simulink model "Ld_Lq_realised_inverter"  (R2024a)
settings: Solver=ode23tb  StartTime=0.0  StopTime=0.25  MaxStep=1e-7  RelTol=1e-3  EnableMultiTasking=on
undefined symbols (not defined in the file): sigbuilder_block
libraries: spsSeriesRLCBranchLib x8, spsVoltageMeasurementLib x8, spsIGBTDiodeLib x6, spsRMSLib x4, spsCurrentMeasurementLib x3, spsMeanLib x3, simulink x3, spsPermanentMagnetSynchronousMachineLib x1, spsThreePhaseSourceLib x1, spsUniversalBridgeLib x1, spspowerguiLib x1
settings Model: Creator=Алексей  LastModifiedBy=alexey
settings SolverCC: ZeroCrossControl=DisableAll  ZeroCrossAlgorithm=Adaptive  AlgebraicLoopSolver=TrustRegion
settings DataIOCC: SaveFormat=Array  SaveOutput=off  SignalLogging=off  DSMLogging=off  SaveTime=off  ReturnWorkspaceOutputs=off
settings OptimizationCC: LifeSpan=inf
settings DebuggingCC: UnderspecifiedInitializationDetection=Classic  MergeDetectMultiDrivingBlocksExec=none  SolverPrmCheckMsg=warning  UnconnectedInputMsg=warning  UnconnectedOutputMsg=warning  UnconnectedLineMsg=warning  AllowSymbolicDim=off  SFUnexpectedBacktrackingDiag=warning  SFNoUnconditionalDefaultTransitionDiag=warning  SFExecutionAtInitializationDiag=none  ArithmeticOperatorsInVariantConditions=warning
settings HardwareCC: ProdBitPerPointer=32  ProdBitPerSizeT=32  ProdBitPerPtrDiffT=32  ProdLargestAtomicFloat=None  ProdIntDivRoundTo=Undefined  ProdEndianess=Unspecified  ProdWordSize=32  ProdHWDeviceType=32-bit Generic
settings ModelReferenceCC: EnableRefExpFcnMdlSchedulingChecks=on  PropagateSignalLabelsOutOfModel=off
settings SFSimCC: SimUseLocalCustomCode=off  CustomCodeUndefinedFunction=UseInterfaceOnly
settings RTWCC: RTWUseLocalCustomCode=off  GPUComputeCapability=3.5  DLArmComputeVersion=19.05
settings CodeAppCC: StateflowObjectComments=on
settings GRTTargetCC: TargetLangStandard=C89/C90 (ANSI)  RTWCAPISignals=on  RTWCAPIParams=on
settings ConfigComp: CovMetricSettings=dw  CovSaveCumulativeToWorkspaceVar=on  CovSaveSingleToWorkspaceVar=on  CovExternalEMLEnable=off  CovSFcnEnable=off
settings SimscapeCC: SimscapeNormalizeSystem=off

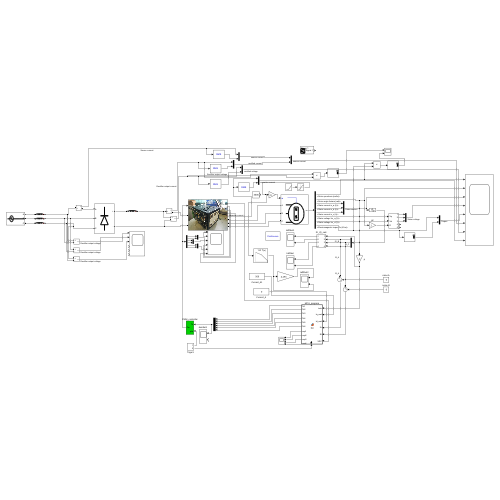
[thumbnail: Simulink's stored preview of the top-level diagram]
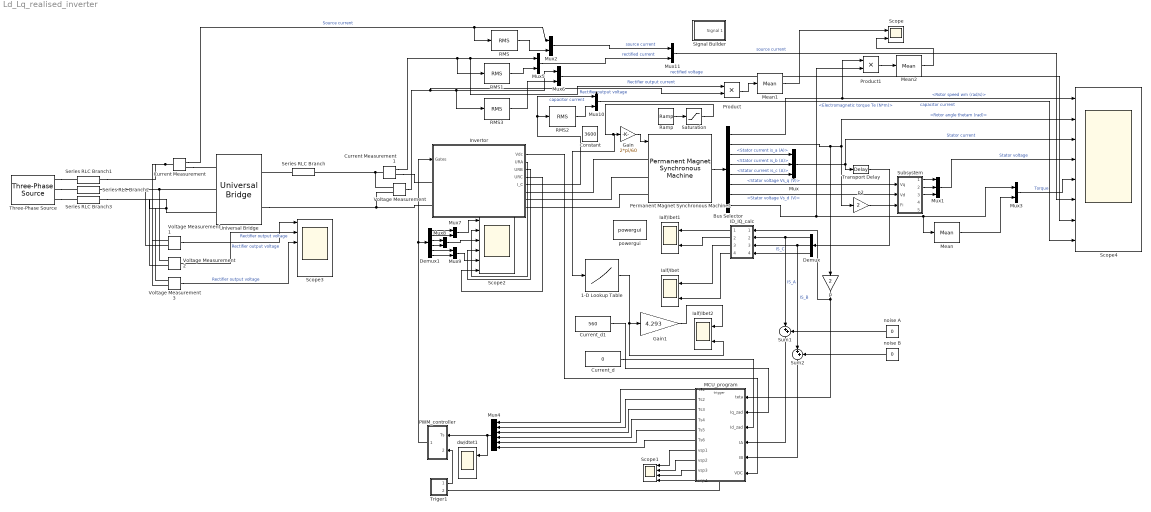
== system Ld_Lq_realised_inverter ==
  1-D Lookup Table : Lookup_n-D  NumberOfTableDimensions=1  BreakpointsForDimension1=[0 2834 5667 5668 5669]  Table=[140 105 25 0 0]  InternalRulePriority=Speed  RndMeth=Simplest
  Bus Selector : BusSelector  OutputSignals=Rotor speed wm (rad/s),Rotor angle thetam (rad),Stator current is_a (A),Stator current is_b (A),Stator current is_c (A),Stator voltage Vs_q (V),Stator voltage Vs_d (V),Electromagnetic torque Te (N*m)
  Constant : Constant  Value=3600
  Current Measurement : spsCurrentMeasurementLib/Current Measurement  PhasorSimulation=off  OutputType=Complex  PSBequivalent=0
  Current Measurement1 : spsCurrentMeasurementLib/Current Measurement  PhasorSimulation=off  OutputType=Complex  PSBequivalent=0
  Current_d : Constant  Value=0
  Current_d1 : Constant  Value=560
  Demux : Demux  Outputs=3
  Demux1 : Demux  Outputs=6
  Gain : Gain  Gain=2*pi/60
  Gain1 : Gain  Gain=4.293
  ID_IQ_calc : Subsystem
  Ialf/Ibet : Scope  NumInputPorts=2
  Ialf/Ibet1 : Scope  NumInputPorts=2
  Ialf/Ibet2 : Scope  NumInputPorts=2
  Invertor : Subsystem
      mask Display: image('$imagefile'); % Use "Edit Image" on toolstrip to change.
  MCU_program : MATLAB Function  TreatAsAtomicUnit=on
  Mean : spsMeanLib/Mean  Freq=1000  Vinit=0  Ts=0
  Mean1 : spsMeanLib/Mean  Freq=400  Vinit=0  Ts=0
  Mean2 : spsMeanLib/Mean  Freq=400  Vinit=0  Ts=0
  Mux : Mux  Inputs=3
  Mux1 : Mux  Inputs=3
  Mux{2..3,5..11} (9 alike) : Mux  Inputs=2
  Mux4 : Mux  Inputs=6
  PWM_controller : Subsystem
  Permanent Magnet Synchronous Machine1 : spsPermanentMagnetSynchronousMachineLib/Permanent Magnet Synchronous Machine  NbPhases=3  FluxDistribution=Sinusoidal  RotorType=Round  MechanicalLoad=Speed w  PresetModel=No  ShowDetailedParameters=on  MeasurementBus=off  Resistance=0.00285  Inductance=8.5e-3  dqInductances=[0.37e-3, 1.075e-3]  La=68.03e-6  MachineConstant=Flux linkage established by magnets (V.s)  Flux=0.07763  VoltageCst=28.161  TorqueCst=0.23289  Flat=120  Mechanical=[2e104 3e-03 2 0]  PolePairs=2  InitialConditions=[0,0, 0,0]  InitialConditions5ph=[0 0 0 0 0 0]  RefAngle=Aligned with phase A axis (original Park)  IterativeDiscreteModel=Trapezoidal non iterative  TsBlock=-1  TsPowergui=0
  Product : Product
  Product1 : Product
  RMS : spsRMSLib/RMS  TrueRMS=on  Freq=400  RMSInit=120  Ts=0
  RMS1 : spsRMSLib/RMS  TrueRMS=on  Freq=400  RMSInit=120  Ts=0
  RMS2 : spsRMSLib/RMS  TrueRMS=on  Freq=400  RMSInit=120  Ts=0
  RMS3 : spsRMSLib/RMS  TrueRMS=on  Freq=400  RMSInit=280  Ts=0
  Ramp : simulink/Sources/Ramp  slope=36000  start=0.01  InitialOutput=0
  Saturation : Saturate  UpperLimit=5600
  Scope : Scope  NumInputPorts=2
  Scope1 : Scope  NumInputPorts=4
  Scope2 : Scope  NumInputPorts=6
  Scope3 : Scope  NumInputPorts=6
  Scope4 : Scope  NumInputPorts=8
  Series RLC Branch : spsSeriesRLCBranchLib/Series RLC Branch  LConnTagsString=__new0  RConnTagsString=__new0  BranchType=L  Resistance=1  Inductance=15e-6  SetiL0=off  InitialCurrent=0  Capacitance=1000e-6  Setx0=on  InitialVoltage=282  Measurements=None
  Series RLC Branch1 : spsSeriesRLCBranchLib/Series RLC Branch  LConnTagsString=__new0  RConnTagsString=__new0  BranchType=L  Resistance=1  Inductance=50e-9  SetiL0=off  InitialCurrent=0  Capacitance=1000e-6  Setx0=on  InitialVoltage=282  Measurements=None
  Series RLC Branch2 : spsSeriesRLCBranchLib/Series RLC Branch  LConnTagsString=__new0  RConnTagsString=__new0  BranchType=L  Resistance=1  Inductance=50e-9  SetiL0=off  InitialCurrent=0  Capacitance=1000e-6  Setx0=on  InitialVoltage=282  Measurements=None
  Series RLC Branch3 : spsSeriesRLCBranchLib/Series RLC Branch  LConnTagsString=__new0  RConnTagsString=__new0  BranchType=L  Resistance=1  Inductance=50e-9  SetiL0=off  InitialCurrent=0  Capacitance=1000e-6  Setx0=on  InitialVoltage=282  Measurements=None
  Signal Builder : Subsystem  Tag=STV Subsys  LoadFcn=sigbuilder_block('load');  StartFcn=sigbuilder_block('start');  StopFcn=sigbuilder_block('stop');  ClipboardFcn=sigbuilder_block('clipboard');  mask(Sigbuilder block){tuvar=[0:10]}
      mask help: Simulink:masks:SigbuilderBlock_MD
      mask init:
      | if ~strcmp(get_param(bdroot(gcbh),'SimulationStatus'),'stopped') tuvar = sigbuilder_block('maskInit'); end
      settings: CopyFcn=sigbuilder_block('copy');  DeleteFcn=sigbuilder_block('delete');  ModelCloseFcn=sigbuilder_block('modelClose');  PreSaveFcn=sigbuilder_block('preSave');  PauseFcn=sigbuilder_block('pause');  ContinueFcn=sigbuilder_block('continue');  NameChangeFcn=sigbuilder_block('namechange');  OpenFcn=sigbuilder_block('open',[60 199.2 1136.8 400 ]);  CloseFcn=sigbuilder_block('close');
      mask Display: plot(0, 0, 100, 100,[2, 2, 32, 32, 2], [68, 8, 8, 68, 68],[32, 2], [38, 38], [32, 19, 2],[53, 60, 44], [32, 17, 17, 2],[16, 16, 31, 31]);txt = getActiveGroup(gcbh);text(2, 100, txt,'verticalAlignment', 'top');
  Subsystem : Subsystem
  Sum1 : Sum  Inputs=|++
  Sum2 : Sum  Inputs=|++
  Three-Phase Source : spsThreePhaseSourceLib/Three-Phase Source  InternalConnection=Y  VoltagePhases=off  Voltage=200  PhaseAngle=0  Voltage_phases=[25e3 25e3 25e3]/sqrt(3)  PhaseAngles_phases=[0 -120 +120]  Frequency=400  NonIdealSource=off  SpecifyImpedance=off  Resistance=0.02e-3  Inductance=30e-9  ShortCircuitLevel=100e6  BaseVoltage=200  XRratio=7  BusType=swing  Pref=10e3  Qref=0  Prefabc=[10e3, 10e3, 10e3]  Qrefabc=[0, 0, 0]  Qmin=-inf  Qmax=inf
  Transport Delay : TransportDelay  DelayTime=5e-6
  Triger1 : Subsystem
  Universal Bridge : spsUniversalBridgeLib/Universal Bridge  Arms=3  SnubberResistance=1e5  SnubberCapacitance=inf  Device=Diodes  Ron=1e-3  Lon=0  ForwardVoltages="[  0  0  ]"  ForwardVoltage=0  GTOparameters=[ 10e-6 , 20e-6 ]  IGBTparameters=[ 1e-6 , 2e-6 ]  Measurements=None  Measurements_2=None  converterType=Rectifier
  Voltage Measurement{,1..3} (4 alike) : spsVoltageMeasurementLib/Voltage Measurement  PhasorSimulation=off  OutputType=Complex  PSBequivalent=0
  dw/dtet1 : Scope  NumInputPorts=2
  noise A : Constant  Value=0
  noise B : Constant  Value=0
  p : Gain  Gain=2
  p2 : Gain  Gain=2
  powergui : spspowerguiLib/powergui  Priority=1  SimulationMode=Continuous  SampleTime=50e-6  frequency=60  Iterations=50  frequencyindice=0  Pbase=100e6  ErrMax=1e-4  UnitsV=kV  UnitsW=MW  buscounter=0  FunctionMessages=off  echomessages=off  EnableUseOfTLC=off  CurrentSourceSwitches=on  DisableSnubberDevices=off  DisableRonSwitches=off  DisableVfSwitches=off  DisplayEquations=off  AutomaticDiscreteSolvers=off  SolverType=Tustin  Interpol=off  ExternalGateDelay=off  methode=off  Ts=0  x0status=blocks  SPID=off  SwTol=0  HookPort=off  NonlinearTolerance=1e-4  nMaxIteration=100  ContinueOnMaxIteration=off  RestoreLinks=warning  ResistiveCurrentMeasurement=off  Frange=[0:2:500]  Ylog=off  Xlog=on  ShowGrid=off  save=off  variable=ZData  structure=SD2  ZoomFFT=on  StartTime=0.7  cycles=10  DisplayStyle=4  fundamental=382  FreqAxis=off  MaxFrequency=50000  frequencyindicesteady=1  RmsSteady=1  display=off
  wires:
  Demux/1 -> ID_IQ_calc/2(In2), Sum1/1  "IS_A"
  Demux/2 -> ID_IQ_calc/3(In3), Sum2/1  "IS_B"
  Permanent Magnet Synchronous Machine1/1 -> Bus Selector/1
  Bus Selector/3 -> Mux/1  "<Stator current is_a (A)>"
  Bus Selector/4 -> Mux/2  "<Stator current is_b (A)>"
  Bus Selector/5 -> Mux/3  "<Stator current is_c (A)>"
  Bus Selector/6 -> Subsystem/1(Vq)  "<Stator voltage Vs_q (V)>"
  Bus Selector/7 -> Subsystem/2(Vd)  "<Stator voltage Vs_d (V)>"
  Subsystem/2(Out2) -> Mux1/2
  Subsystem/3(Out3) -> Mux1/3
  Subsystem/1(Out1) -> Mux1/1
  Mux/1 -> Scope4/3, Transport Delay/1  "Stator current"
  Mux1/1 -> Scope4/4  "Stator voltage"
  Bus Selector/8 -> Product1/2, Mean/1, Mux3/1  "<Electromagnetic torque Te (N*m)>"
  Demux/3 -> ID_IQ_calc/4(In4)  "IS_C"
  Gain/1 -> Permanent Magnet Synchronous Machine1/1
  MCU_program/8(vsp2) -> Scope1/2
  MCU_program/9(vsp3) -> Scope1/3
  MCU_program/7(vsp1) -> Scope1/1
  Sum1/1 -> MCU_program/4(IA)
  Sum2/1 -> MCU_program/5(IB)
  Bus Selector/1 -> Product1/1, Scope4/1  "<Rotor speed wm (rad/s)>"
  Bus Selector/2 -> p2/1, Scope4/2, p/1  "<Rotor angle thetam (rad)>"
  Transport Delay/1 -> Demux/1
  noise A/1 -> Sum1/2
  noise B/1 -> Sum2/2
  MCU_program/10(vsp4) -> Scope1/4
  ID_IQ_calc/3(Out3) -> Ialf/Ibet/1
  ID_IQ_calc/4(Out4) -> Ialf/Ibet/2
  p/1 -> MCU_program/1(teta), ID_IQ_calc/1(In1)
  p2/1 -> Subsystem/3(Fi)
  Gain1/1 -> Ialf/Ibet2/1
  Current_d/1 -> MCU_program/3(Id_zad)
  ID_IQ_calc/1(Out1) -> Ialf/Ibet1/1
  ID_IQ_calc/2(Out2) -> Ialf/Ibet1/2
  Mux3/1 -> Scope4/5  "Torque"
  Mean/1 -> Mux3/2
  Demux1/6 -> Mux9/2
  MCU_program/6(Ts6) -> Mux4/6
  MCU_program/5(Ts5) -> Mux4/5
  Demux1/1 -> Mux7/1
  MCU_program/4(Ts4) -> Mux4/4
  Invertor/3(URB) -> Scope2/4
  Demux1/5 -> Mux9/1
  Demux1/4 -> Mux8/2
  MCU_program/3(Ts3) -> Mux4/3
  Triger1/1(1) -> PWM_controller/2(pila)
  Mux9/1 -> Scope2/5
  PWM_controller/1(Tss) -> Invertor/1(Gates), Demux1/1
  Mux7/1 -> Scope2/1
  Demux1/2 -> Mux7/2
  MCU_program/1(Ts1) -> Mux4/1
  Mux4/1 -> dw/dtet1/1, PWM_controller/1(Ts)
  Triger1/2(2) -> MCU_program/Trigger
  MCU_program/2(Ts2) -> Mux4/2
  Invertor/2(URA) -> Scope2/2
  Demux1/3 -> Mux8/1
  Mux8/1 -> Scope2/3
  Invertor/4(URC) -> Scope2/6
  Invertor/1(Vdc) -> MCU_program/6(VDC)
  Invertor/5(I_C) -> RMS2/1, Mux10/1  "capacitor current"
  Current Measurement/1 -> RMS/1, Mux2/1  "Source current"
  Current Measurement1/1 -> RMS1/1, Product/1, Mux5/1  "Rectifier output current"
  Voltage Measurement/1 -> Product/2, RMS3/1, Mux6/1  "Rectifier output voltage"
  Mux2/1 -> Mux11/1  "source current"
  RMS/1 -> Mux2/2
  Mux5/1 -> Mux11/2  "rectified current"
  Mux6/1 -> Scope4/7  "rectified voltage"
  RMS1/1 -> Mux5/2
  RMS2/1 -> Mux10/2
  Mux10/1 -> Scope4/8  "capacitor current"
  RMS3/1 -> Mux6/2
  Saturation/1 -> 1-D Lookup Table/1, Gain/1
  1-D Lookup Table/1 -> Ialf/Ibet2/2, Gain1/1
  Mux11/1 -> Scope4/6  "source current"
  Current_d1/1 -> MCU_program/2(Iq_zad)
  Ramp/1 -> Saturation/1
  Voltage Measurement1/1 -> Scope3/1  "Rectifier output voltage"
  Voltage Measurement2/1 -> Scope3/2  "Rectifier output voltage"
  Voltage Measurement3/1 -> Scope3/3  "Rectifier output voltage"
  Product/1 -> Mean1/1
  Mean1/1 -> Scope/1
  Product1/1 -> Mean2/1
  Mean2/1 -> Scope/2
  connections:
  Permanent Magnet Synchronous Machine1/LConn1 -- Invertor/RConn1
  Permanent Magnet Synchronous Machine1/LConn3 -- Invertor/RConn3
  Permanent Magnet Synchronous Machine1/LConn2 -- Invertor/RConn2
  Current Measurement/LConn1 -- Series RLC Branch1/LConn1 -- Voltage Measurement1/LConn1 -- Voltage Measurement3/LConn2
  Series RLC Branch2/LConn1 -- Voltage Measurement1/LConn2 -- Voltage Measurement2/LConn1 -- Universal Bridge/LConn2
  Series RLC Branch3/LConn1 -- Voltage Measurement2/LConn2 -- Voltage Measurement3/LConn1 -- Universal Bridge/LConn3
  Current Measurement1/RConn1 -- Invertor/LConn1
  Universal Bridge/RConn2 -- Voltage Measurement/LConn2 -- Invertor/LConn2
  Current Measurement/RConn1 -- Universal Bridge/LConn1
  Series RLC Branch/RConn1 -- Universal Bridge/RConn1
  Current Measurement1/LConn1 -- Voltage Measurement/LConn1 -- Series RLC Branch/LConn1
  Three-Phase Source/RConn1 -- Series RLC Branch1/RConn1
  Three-Phase Source/RConn2 -- Series RLC Branch2/RConn1
  Three-Phase Source/RConn3 -- Series RLC Branch3/RConn1

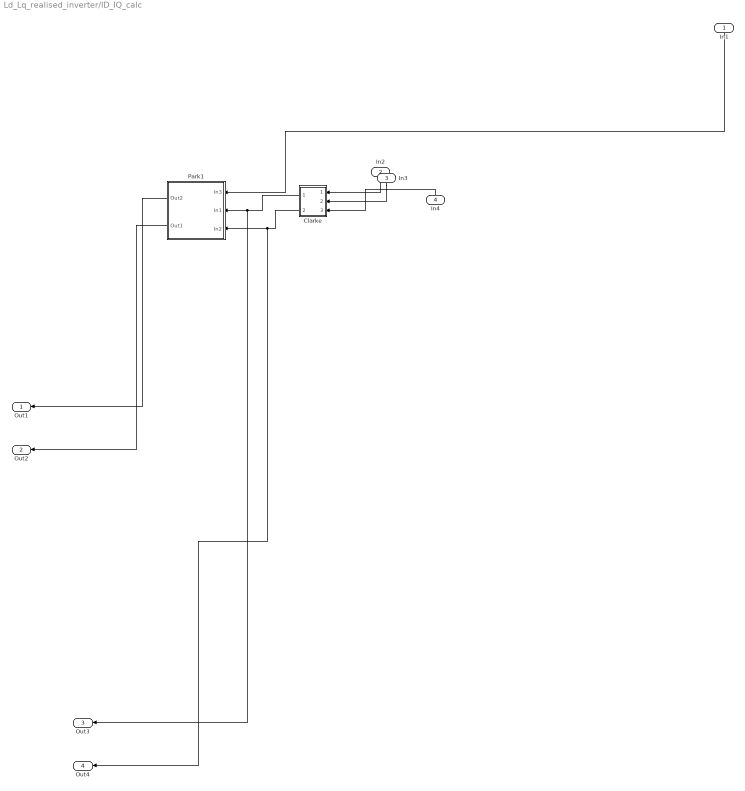
== system Ld_Lq_realised_inverter/ID_IQ_calc ==
  In1 : Inport
  In2 : Inport  Port=2
  In3 : Inport  Port=3
  In4 : Inport  Port=4
  Clarke : Subsystem
  Park1 : Subsystem
  Out1 : Outport  VectorParamsAs1DForOutWhenUnconnected=off
  Out2 : Outport  Port=2  VectorParamsAs1DForOutWhenUnconnected=off
  Out3 : Outport  Port=3  VectorParamsAs1DForOutWhenUnconnected=off
  Out4 : Outport  Port=4  VectorParamsAs1DForOutWhenUnconnected=off
  wires:
  Park1/2(Out1) -> Out2/1
  Park1/1(Out2) -> Out1/1
  In1/1 -> Park1/1(In3)
  In4/1 -> Clarke/3(In3)
  In2/1 -> Clarke/1(In1)
  In3/1 -> Clarke/2(In2)
  Clarke/2(Out1) -> Out4/1, Park1/3(In2)
  Clarke/1(Out2) -> Out3/1, Park1/2(In1)

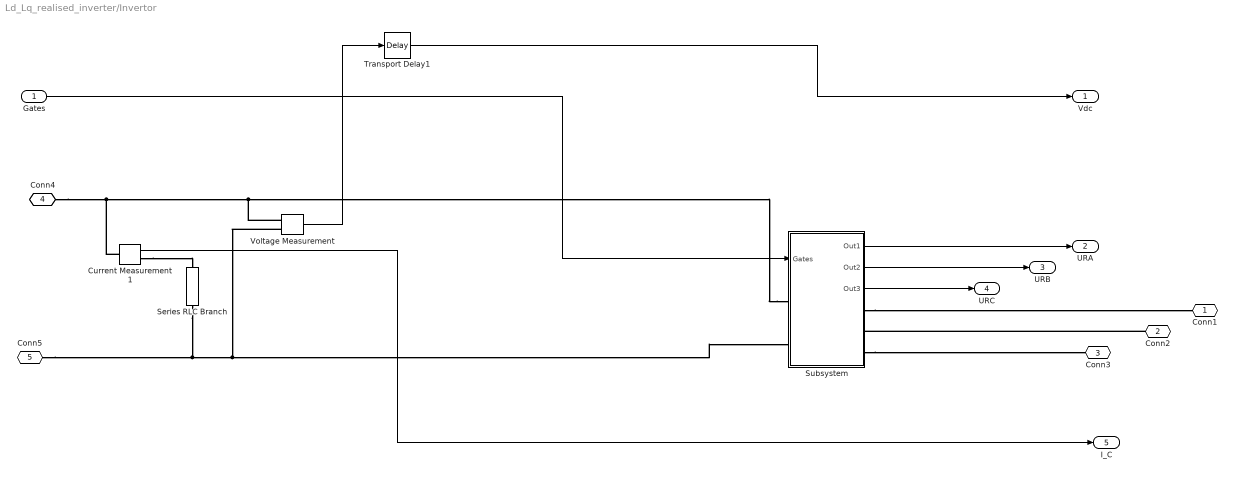
== system Ld_Lq_realised_inverter/Invertor ==
  Gates : Inport
  Current Measurement1 : spsCurrentMeasurementLib/Current Measurement  PhasorSimulation=off  OutputType=Complex  PSBequivalent=0
  Series RLC Branch : spsSeriesRLCBranchLib/Series RLC Branch  LConnTagsString=__new0  RConnTagsString=__new0  BranchType=C  Resistance=1  Inductance=1e-3  SetiL0=off  InitialCurrent=0  Capacitance=4000e-6  Setx0=on  InitialVoltage=282  Measurements=None
  Subsystem : Subsystem
  Transport Delay1 : TransportDelay  DelayTime=26e-6
  Voltage Measurement : spsVoltageMeasurementLib/Voltage Measurement  PhasorSimulation=off  OutputType=Complex  PSBequivalent=0
  Conn1 : PMIOPort  Side=Right
  Conn2 : PMIOPort  Port=2  Side=Right
  Conn3 : PMIOPort  Port=3  Side=Right
  Conn4 : PMIOPort  Port=4  Side=Left
  Conn5 : PMIOPort  Port=5  Side=Left
  Vdc : Outport  VectorParamsAs1DForOutWhenUnconnected=off
  URA : Outport  Port=2  VectorParamsAs1DForOutWhenUnconnected=off
  URB : Outport  Port=3  VectorParamsAs1DForOutWhenUnconnected=off
  URC : Outport  Port=4  VectorParamsAs1DForOutWhenUnconnected=off
  I_C : Outport  Port=5  VectorParamsAs1DForOutWhenUnconnected=off
  wires:
  Voltage Measurement/1 -> Transport Delay1/1
  Transport Delay1/1 -> Vdc/1
  Gates/1 -> Subsystem/1(Gates)
  Subsystem/1(Out1) -> URA/1
  Subsystem/2(Out2) -> URB/1
  Subsystem/3(Out3) -> URC/1
  Current Measurement1/1 -> I_C/1
  connections:
  Subsystem/LConn1 -- Current Measurement1/LConn1 -- Conn4/RConn1 -- Voltage Measurement/LConn1
  Voltage Measurement/LConn2 -- Series RLC Branch/RConn1 -- Conn5/RConn1 -- Subsystem/LConn2
  Subsystem/RConn1 -- Conn1/RConn1
  Conn2/RConn1 -- Subsystem/RConn2
  Subsystem/RConn3 -- Conn3/RConn1
  Current Measurement1/RConn1 -- Series RLC Branch/LConn1

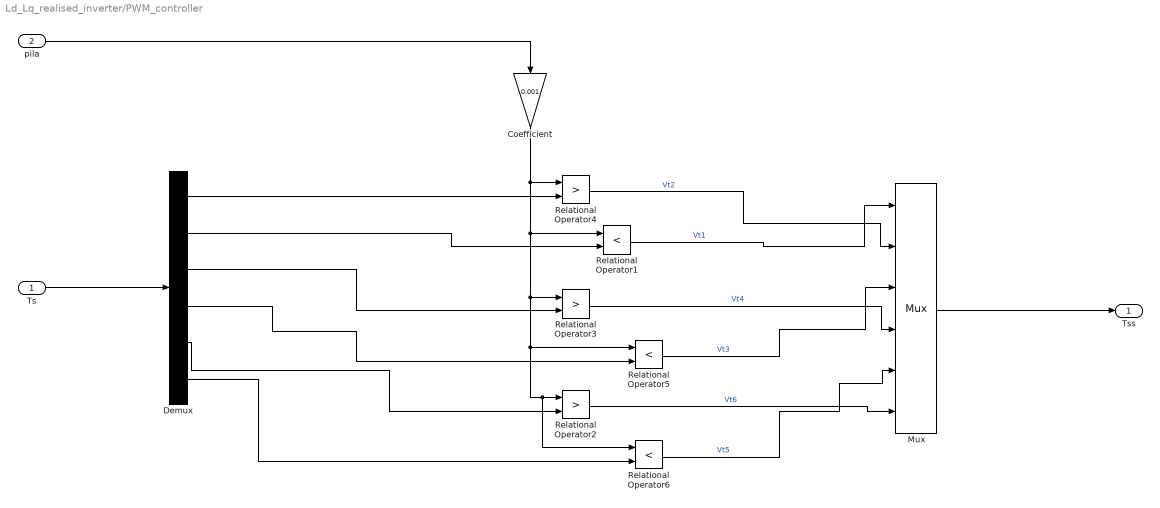
== system Ld_Lq_realised_inverter/PWM_controller ==
  Ts : Inport
  pila : Inport  Port=2
  Coefficient : Gain  Gain=0.001
  Demux : Demux  Outputs=6
  Mux : Mux  Inputs=6
  Relational Operator1 : RelationalOperator  Operator=<  OutDataTypeStr=boolean  InputSameDT=off
  Relational Operator2 : RelationalOperator  Operator=>  OutDataTypeStr=boolean  InputSameDT=off
  Relational Operator3 : RelationalOperator  Operator=>  OutDataTypeStr=boolean  InputSameDT=off
  Relational Operator4 : RelationalOperator  Operator=>  OutDataTypeStr=boolean  InputSameDT=off
  Relational Operator5 : RelationalOperator  Operator=<  OutDataTypeStr=boolean  InputSameDT=off
  Relational Operator6 : RelationalOperator  Operator=<  OutDataTypeStr=boolean  InputSameDT=off
  Tss : Outport  VectorParamsAs1DForOutWhenUnconnected=off
  wires:
  Relational Operator4/1 -> Mux/2  "Vt2"
  Demux/3 -> Relational Operator3/2
  Demux/5 -> Relational Operator2/2
  Relational Operator3/1 -> Mux/4  "Vt4"
  Relational Operator2/1 -> Mux/6  "Vt6"
  Ts/1 -> Demux/1
  Coefficient/1 -> Relational Operator1/1, Relational Operator3/1, Relational Operator5/1, Relational Operator6/1, Relational Operator2/1, Relational Operator4/1
  Relational Operator1/1 -> Mux/1  "Vt1"
  Relational Operator5/1 -> Mux/3  "Vt3"
  Relational Operator6/1 -> Mux/5  "Vt5"
  Demux/2 -> Relational Operator1/2
  Demux/4 -> Relational Operator5/2
  Demux/6 -> Relational Operator6/2
  Demux/1 -> Relational Operator4/2
  pila/1 -> Coefficient/1
  Mux/1 -> Tss/1

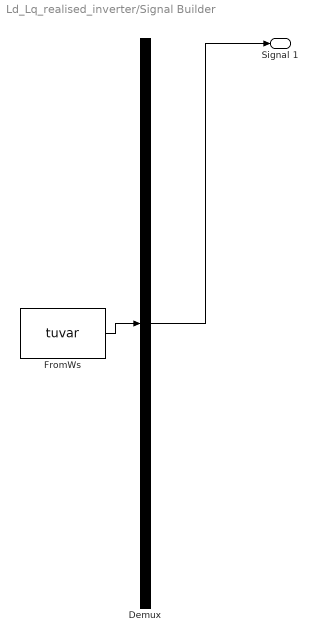
== system Ld_Lq_realised_inverter/Signal Builder ==
  Demux : Demux  Tag=STV Demux  Outputs=1
      settings: DisplayOption=none
  FromWs : FromWorkspace  Tag=STV FromWs  VariableName=tuvar
      SigBuilderData=|
      | common.afterFinalStr = 'Extrapolate'
      | common.sampleTime = 0
      | dataSet.timeRange = [0 40]
      | dataSet.name = 'Group 1'
      | sbobj.Groups.Name = 'Group 1'
      | sbobj.Groups.Signals.Name = 'Signal 1'
      | sbobj.Groups.Signals.XData = [0 0.15 0.35 40]
      | sbobj.Groups.Signals.YData = [0 2834 5667 11000]
      | sbobj.Groups.TimeRange = [0 40]
  Signal 1 : Outport  Tag=STV Outport
  wires:
  Demux/1 -> Signal 1/1
  FromWs/1 -> Demux/1

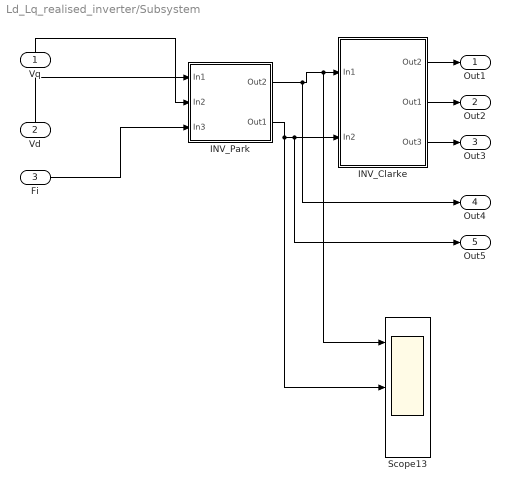
== system Ld_Lq_realised_inverter/Subsystem ==
  Vq : Inport
  Vd : Inport  Port=2
  Fi : Inport  Port=3
  INV_Clarke : Subsystem
  INV_Park : Subsystem
  Scope13 : Scope  NumInputPorts=3
  Out1 : Outport  VectorParamsAs1DForOutWhenUnconnected=off
  Out2 : Outport  Port=2  VectorParamsAs1DForOutWhenUnconnected=off
  Out3 : Outport  Port=3  VectorParamsAs1DForOutWhenUnconnected=off
  Out4 : Outport  Port=4  VectorParamsAs1DForOutWhenUnconnected=off
  Out5 : Outport  Port=5  VectorParamsAs1DForOutWhenUnconnected=off
  wires:
  INV_Clarke/2(Out1) -> Out2/1
  INV_Park/1(Out2) -> Out4/1, Scope13/1, INV_Clarke/1(In1)
  INV_Clarke/1(Out2) -> Out1/1
  INV_Park/2(Out1) -> Scope13/2, Out5/1, INV_Clarke/2(In2)
  INV_Clarke/3(Out3) -> Out3/1
  Fi/1 -> INV_Park/3(In3)
  Vd/1 -> INV_Park/1(In1)
  Vq/1 -> INV_Park/2(In2)

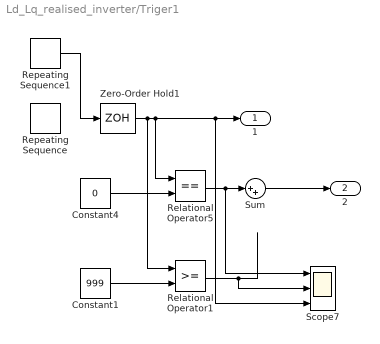
== system Ld_Lq_realised_inverter/Triger1 ==
  Constant1 : Constant  Value=999
  Constant4 : Constant  Value=0
  Relational Operator1 : RelationalOperator  OutDataTypeStr=boolean  InputSameDT=off
  Relational Operator5 : RelationalOperator  Operator===  OutDataTypeStr=boolean  InputSameDT=off
  Repeating Sequence : simulink/Sources/Repeating Sequence  rep_seq_t=[0 10e-5]  rep_seq_y=[0 1000]
  Repeating Sequence1 : simulink/Sources/Repeating Sequence  rep_seq_t=[0 5e-5 10e-5]  rep_seq_y=[0 1000 0]
  Scope7 : Scope  NumInputPorts=3
  Sum : Sum  Inputs=|++
  Zero-Order Hold1 : ZeroOrderHold  SampleTime=5e-8
  1 : Outport  VectorParamsAs1DForOutWhenUnconnected=off
  2 : Outport  Port=2  VectorParamsAs1DForOutWhenUnconnected=off
  wires:
  Zero-Order Hold1/1 -> Relational Operator1/1, Relational Operator5/1, Scope7/3, 1/1
  Repeating Sequence1/1 -> Zero-Order Hold1/1
  Constant4/1 -> Relational Operator5/2
  Sum/1 -> 2/1
  Constant1/1 -> Relational Operator1/2
  Relational Operator5/1 -> Scope7/1, Sum/1
  Relational Operator1/1 -> Scope7/2

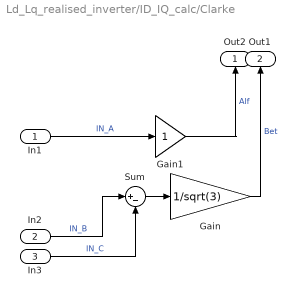
== system Ld_Lq_realised_inverter/ID_IQ_calc/Clarke ==
  In1 : Inport
  In2 : Inport  Port=2
  In3 : Inport  Port=3
  Gain : Gain  Gain=1/sqrt(3)
  Gain1 : Gain
  Sum : Sum  Inputs=|+-
  Out2 : Outport  VectorParamsAs1DForOutWhenUnconnected=off
  Out1 : Outport  Port=2  VectorParamsAs1DForOutWhenUnconnected=off
  wires:
  Gain/1 -> Out1/1  "Bet"
  In2/1 -> Sum/1  "IN_B"
  In1/1 -> Gain1/1  "IN_A"
  In3/1 -> Sum/2  "IN_C"
  Sum/1 -> Gain/1
  Gain1/1 -> Out2/1  "Alf"

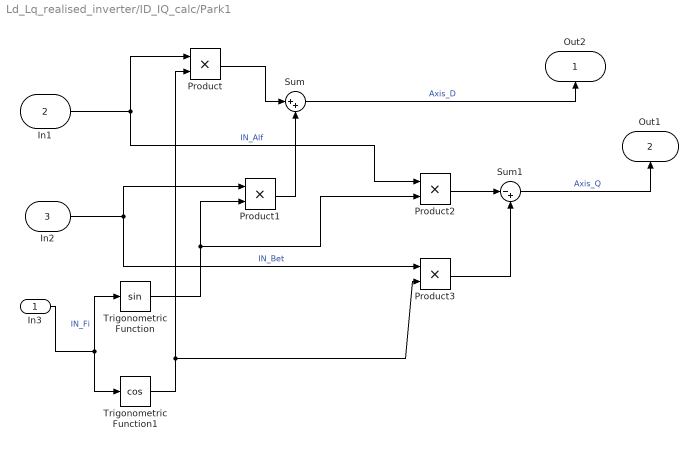
== system Ld_Lq_realised_inverter/ID_IQ_calc/Park1 ==
  In3 : Inport
  In1 : Inport  Port=2
  In2 : Inport  Port=3
  Product{,1..3} (4 alike) : Product
  Sum : Sum  Inputs=|++
  Sum1 : Sum  Inputs=|-+
  Trigonometric Function : Trigonometry
  Trigonometric Function1 : Trigonometry  Operator=cos
  Out2 : Outport  VectorParamsAs1DForOutWhenUnconnected=off
  Out1 : Outport  Port=2  VectorParamsAs1DForOutWhenUnconnected=off
  wires:
  Sum1/1 -> Out1/1  "Axis_Q"
  In2/1 -> Product1/1, Product3/1  "IN_Bet"
  In1/1 -> Product2/1, Product/1  "IN_Alf"
  Sum/1 -> Out2/1  "Axis_D"
  In3/1 -> Trigonometric Function1/1, Trigonometric Function/1  "IN_Fi"
  Trigonometric Function1/1 -> Product/2, Product3/2
  Trigonometric Function/1 -> Product2/2, Product1/2
  Product1/1 -> Sum/2
  Product/1 -> Sum/1
  Product2/1 -> Sum1/1
  Product3/1 -> Sum1/2

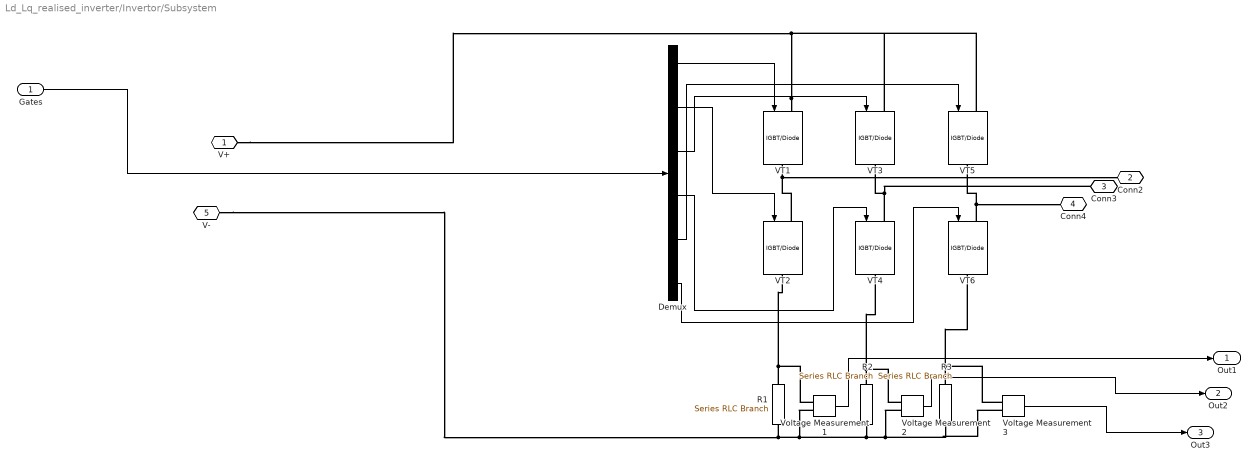
== system Ld_Lq_realised_inverter/Invertor/Subsystem ==
  Gates : Inport
  Demux : Demux  Outputs=6
  R1 : spsSeriesRLCBranchLib/Series RLC Branch  LConnTagsString=__new0  RConnTagsString=__new0  BranchType=R  Resistance=0.001  Inductance=1e-3  SetiL0=off  InitialCurrent=0  Capacitance=30e-6  Setx0=on  InitialVoltage=220  Measurements=None
  R2 : spsSeriesRLCBranchLib/Series RLC Branch  LConnTagsString=__new0  RConnTagsString=__new0  BranchType=R  Resistance=0.001  Inductance=1e-3  SetiL0=off  InitialCurrent=0  Capacitance=30e-6  Setx0=on  InitialVoltage=220  Measurements=None
  R3 : spsSeriesRLCBranchLib/Series RLC Branch  LConnTagsString=__new0  RConnTagsString=__new0  BranchType=R  Resistance=0.001  Inductance=1e-3  SetiL0=off  InitialCurrent=0  Capacitance=30e-6  Setx0=on  InitialVoltage=220  Measurements=None
  VT{1..6} (6 alike) : spsIGBTDiodeLib/IGBT//Diode  Ron=1e-3  Rs=1e5  Cs=inf  Measurements=off
  Voltage Measurement1 : spsVoltageMeasurementLib/Voltage Measurement  PhasorSimulation=off  OutputType=Complex  PSBequivalent=0
  Voltage Measurement2 : spsVoltageMeasurementLib/Voltage Measurement  PhasorSimulation=off  OutputType=Complex  PSBequivalent=0
  Voltage Measurement3 : spsVoltageMeasurementLib/Voltage Measurement  PhasorSimulation=off  OutputType=Complex  PSBequivalent=0
  V+ : PMIOPort  Side=Left
  Conn2 : PMIOPort  Port=2  Side=Right
  Conn3 : PMIOPort  Port=3  Side=Right
  Conn4 : PMIOPort  Port=4  Side=Right
  V- : PMIOPort  Port=5  Side=Left
  Out1 : Outport  VectorParamsAs1DForOutWhenUnconnected=off
  Out2 : Outport  Port=2  VectorParamsAs1DForOutWhenUnconnected=off
  Out3 : Outport  Port=3  VectorParamsAs1DForOutWhenUnconnected=off
  wires:
  Demux/4 -> VT4/1
  Demux/2 -> VT2/1
  Demux/5 -> VT5/1
  Voltage Measurement2/1 -> Out2/1
  Demux/3 -> VT3/1
  Demux/6 -> VT6/1
  Demux/1 -> VT1/1
  Voltage Measurement3/1 -> Out3/1
  Gates/1 -> Demux/1
  Voltage Measurement1/1 -> Out1/1
  connections:
  VT6/LConn1 -- Conn4/RConn1 -- VT5/RConn1
  R1/LConn1 -- V-/RConn1 -- Voltage Measurement1/LConn2 -- Voltage Measurement3/LConn2 -- R3/LConn1 -- Voltage Measurement2/LConn2 -- R2/LConn1
  R1/RConn1 -- Voltage Measurement1/LConn1 -- VT2/RConn1
  VT4/LConn1 -- Conn3/RConn1 -- VT3/RConn1
  VT1/LConn1 -- V+/RConn1 -- VT5/LConn1 -- VT3/LConn1
  R2/RConn1 -- Voltage Measurement2/LConn1 -- VT4/RConn1
  R3/RConn1 -- Voltage Measurement3/LConn1 -- VT6/RConn1
  VT2/LConn1 -- Conn2/RConn1 -- VT1/RConn1

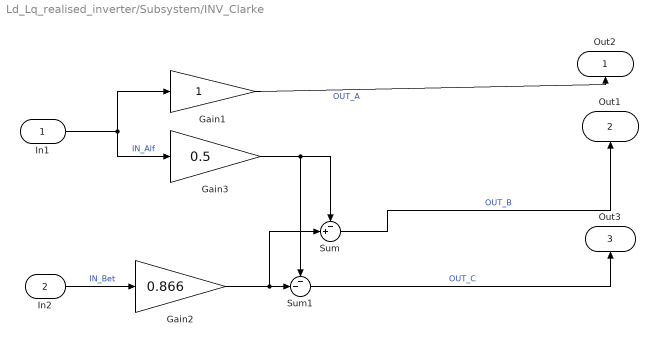
== system Ld_Lq_realised_inverter/Subsystem/INV_Clarke ==
  In1 : Inport
  In2 : Inport  Port=2
  Gain1 : Gain
  Gain2 : Gain  Gain=0.866
  Gain3 : Gain  Gain=0.5
  Sum : Sum  Inputs=-+|
  Sum1 : Sum  Inputs=--|
  Out2 : Outport  VectorParamsAs1DForOutWhenUnconnected=off
  Out1 : Outport  Port=2  VectorParamsAs1DForOutWhenUnconnected=off
  Out3 : Outport  Port=3  VectorParamsAs1DForOutWhenUnconnected=off
  wires:
  Sum/1 -> Out1/1  "OUT_B"
  In2/1 -> Gain2/1  "IN_Bet"
  In1/1 -> Gain1/1, Gain3/1  "IN_Alf"
  Gain1/1 -> Out2/1  "OUT_A"
  Sum1/1 -> Out3/1  "OUT_C"
  Gain3/1 -> Sum1/1, Sum/1
  Gain2/1 -> Sum/2, Sum1/2

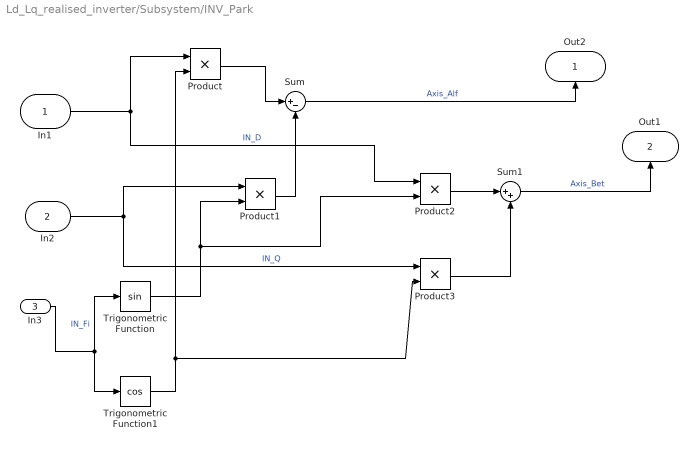
== system Ld_Lq_realised_inverter/Subsystem/INV_Park ==
  In1 : Inport
  In2 : Inport  Port=2
  In3 : Inport  Port=3
  Product{,1..3} (4 alike) : Product
  Sum : Sum  Inputs=|+-
  Sum1 : Sum  Inputs=|++
  Trigonometric Function : Trigonometry
  Trigonometric Function1 : Trigonometry  Operator=cos
  Out2 : Outport  VectorParamsAs1DForOutWhenUnconnected=off
  Out1 : Outport  Port=2  VectorParamsAs1DForOutWhenUnconnected=off
  wires:
  Sum1/1 -> Out1/1  "Axis_Bet"
  In2/1 -> Product1/1, Product3/1  "IN_Q"
  In1/1 -> Product2/1, Product/1  "IN_D"
  Sum/1 -> Out2/1  "Axis_Alf"
  In3/1 -> Trigonometric Function1/1, Trigonometric Function/1  "IN_Fi"
  Trigonometric Function1/1 -> Product/2, Product3/2
  Trigonometric Function/1 -> Product2/2, Product1/2
  Product1/1 -> Sum/2
  Product/1 -> Sum/1
  Product2/1 -> Sum1/1
  Product3/1 -> Sum1/2

== matlab function Ld_Lq_realised_inverter/MCU_program ==
  data: teta input; Iq_zad input; Id_zad input; IA input; IB input; Ts1 output; Ts2 output; Ts3 output; Ts4 output; Ts5 output; Ts6 output; vsp1 output; vsp2 output; vsp3 output; vsp4 output; VDC input
  events: trigger input RISING_EDGE_EVENT
function [Ts1,Ts2,Ts3,Ts4,Ts5,Ts6,vsp1,vsp2,vsp3,vsp4] = fcn(teta,Iq_zad,Id_zad,IA,IB,VDC)
%время 1/2 ШИМ периода
dt=100e-6;

dead_time=0;%0.75

kuqp=1;
kuqi=250;

kudp=1;
kudi=250;





persistent wint;
if isempty(wint)
    wint=0;
end 
persistent Uqint;
if isempty(Uqint)
    Uqint=0;
end 
persistent Udint;
if isempty(Udint)
    Udint=0;
end 


%Преобразование Кларка
Ialfa=IA;
Ibeta=(2*IB+IA)/sqrt(3);
I_ampl=sqrt(Ialfa^2+Ibeta^2);

%реальные значения токов Id и Iq, полученные через  угол и оси альфа,бета 
Id=Ialfa*cos(teta)+Ibeta*sin(teta);
Iq=Ibeta*cos(teta)-Ialfa*sin(teta); 


%ПИ-регулятор для напряжения по оси Ку
diq=Iq_zad-Iq;
Uqpr=diq*kuqp;
Uqint=Uqint+diq*kuqi*dt;

%ПИ-регулятор для напряжения по оси Дэ
did=Id_zad-Id;
Udpr=did*kudp;
Udint=Udint+did*kudi*dt;

Um=(2/3)*VDC/sqrt(Uqpr^2+Udpr^2);

if(Um<1)
  Uqpr=Uqpr*Um;
  Udpr=Udpr*Um;
end

if((Uqpr+Uqint)>0.85*VDC)
  Uqint=0.85*VDC-Uqpr;
end

if(sqrt((Uqpr+Uqint)^2+(Udpr+Udint)^2)>0.85*VDC)
  Udint=sqrt((0.85*VDC)^2-(Uqpr+Uqint)^2)-Udpr;
end
if(Uqint<0)
  Uqint=0;
end
if(Udint<0)
  Udint=0;
end
  
U_q=Uqpr+Uqint;%+1.5*(L*Idr+psi)*wstart%wrez;                    %15.11 поменял omeg на wrez, интересно, как скажется на точности
U_d=Udpr+Udint;%-1.5*(wstart*Iqr*L);   %wrez      %15.11 поменял omeg на wrez, интересно, как скажется на точности

Ua0=U_d*cos(teta)-U_q*sin(teta);
Ub0=U_d*sin(teta)+U_q*cos(teta);

vrefa=sqrt(Ua0^2+Ub0^2);

vphase=acos(Ua0/vrefa)*sign(Ub0)+(sign(Ub0)-1)*(-pi);

if(vrefa>(2/3)*VDC)
  Ua0=Ua0*((2/3)*VDC/vrefa);
  Ub0=Ub0*((2/3)*VDC/vrefa);
end



vsp1=0;
vsp2=0;
vsp3=Id;%wzad-omeg;
vsp4=Iq;


%алгоритм формирования векторной ШИМ  мертвым веменем dead [мкс]

dead_time=dead_time/(dt*1e6);
a=vphase;
v2=vrefa*1.5;
if a>=0 && a<pi/3 
    n=1;
elseif  a>=pi/3 && a<2*pi/3 
    n=2;
elseif  a>=2*pi/3 && a<pi 
    n=3;
elseif  a>=pi && a<4*pi/3 
    n=4;
elseif  a>=4*pi/3 && a<5*pi/3 
    n=5;
else n=6;

end

a_cor=a-(n-1)*pi/3;

T1 = (v2/VDC)*sin(pi/3-a_cor)/sin(pi/3);
T2 = (v2/VDC)*sin(a_cor)/sin(pi/3);
T0=1-T1-T2;
Ta1=0; Ta3=0; Ta5=0; 
switch n
    case 1
        
        Ta1=T1+T2+T0/2;
        
        Ta3=T2+T0/2;
       
        Ta5=T0/2;
       
    case 2
        
        Ta1=T1+T0/2;
        
        Ta3=T1+T2+T0/2;
    
        Ta5=T0/2;       
        
    case 3
        
        Ta1=T0/2;
       
        Ta3=T1+T2+T0/2;
       
        Ta5=T2+T0/2;    
        
    case 4
        
        Ta1=T0/2;
       
        Ta3=T1+T0/2;
       
        Ta5=T1+T2+T0/2;   
       
    case 5
        
        Ta1=T2+T0/2;
        
        Ta3=T0/2;
        
        Ta5=T1+T2+T0/2;     
        
    case 6
        
        Ta1=T1+T2+T0/2;
        
        Ta3=T0/2;
     
        Ta5=T1+T0/2;    
        
end;


Ts1=(Ta1)+dead_time/2; 
Ts3=(Ta3)+dead_time/2; 
Ts5=(Ta5)+dead_time/2;
Ts2=(Ta1)-dead_time/2; 
Ts4=(Ta3)-dead_time/2; 
Ts6=(Ta5)-dead_time/2;


if (IA>0) 
    Ts1=Ts1+dead_time/2;
    Ts2=Ts2+dead_time/2;
else
    Ts1=Ts1-dead_time/2;
    Ts2=Ts2-dead_time/2;           
end;
if (IB>0) 
    Ts3=Ts3+dead_time/2;
    Ts4=Ts4+dead_time/2;
else
    Ts3=Ts3-dead_time/2;
    Ts4=Ts4-dead_time/2; 
end;  
if ((-IA-IB)>0) 
    Ts5=Ts5+dead_time/2;
    Ts6=Ts6+dead_time/2;
else
    Ts5=Ts5-dead_time/2;
    Ts6=Ts6-dead_time/2;           
end;


return;



return;
